simulink model "quad_ndi_test"  (R2017b)
settings: Solver=FixedStepDiscrete  StartTime=0.0  StopTime=10  FixedStep=0.004  RelTol=1e-3
undefined symbols (not defined in the file or in its folder): DiscIntNeverNeededParam
libraries: simulink x3
settings Model: Creator=marcell  LastModifiedBy=max
settings DataIOCC: LimitDataPoints=on
settings OptimizationCC: DefaultParameterBehavior=Inlined  UseFloatMulNetSlope=on  DefaultUnderspecifiedDataType=single  InlineInvariantSignals=on  PassReuseOutputArgsAs=Individual arguments  ZeroExternalMemoryAtStartup=off  ZeroInternalMemoryAtStartup=off  NoFixptDivByZeroProtection=on  EfficientFloat2IntCast=on  LifeSpan=1
settings DebuggingCC: AllowSymbolicDim=off  SFUnexpectedBacktrackingDiag=warning  SFNoUnconditionalDefaultTransitionDiag=warning  SFExecutionAtInitializationDiag=none
settings HardwareCC: ProdBitPerPointer=32  ProdBitPerSizeT=32  ProdBitPerPtrDiffT=32  ProdLargestAtomicInteger=Long  ProdLargestAtomicFloat=Double  ProdWordSize=32  ProdHWDeviceType=ARM Compatible->ARM Cortex
settings ModelReferenceCC: PropagateSignalLabelsOutOfModel=off
settings SFSimCC: MATLABDynamicMemAlloc=off
settings RTWCC: SystemTargetFile=ert.tlc  GenCodeOnly=on  TemplateMakefile=ert_default_tmf  GenerateReport=on  IncludeHyperlinkInReport=on  LaunchReport=on  TargetLang=C++  GenerateTraceInfo=on  GenerateTraceReport=on  GenerateTraceReportSl=on  GenerateTraceReportSf=on  GenerateTraceReportEml=on
settings CodeAppCC: ForceParamTrailComments=on  IgnoreCustomStorageClasses=off  SimulinkDataObjDesc=on  CustomSymbolStrGlobalVar=rt$N$M  CustomSymbolStrType=$N$M  CustomSymbolStrFcn=$N$M$F  CustomSymbolStrMacro=$N$M  InsertBlockDesc=on  StateflowObjectComments=on
settings ERTTargetCC: MultiwordLength=2048  GenerateSampleERTMain=on  IncludeMdlTerminateFcn=off  CombineSignalStateStructs=on  SupportAbsoluteTime=off  MultiInstanceERTCode=on  CodeInterfacePackaging=C++ class  SupportNonFinite=off  SupportComplex=off  SupportNonInlinedSFcns=on  InlinedParameterPlacement=NonHierarchical  RootIOFormat=Structure reference  ERTCustomFileTemplate=example_file_process.tlc  ERTFilePackagingFormat=CompactWithDataFile  ConvertIfToSwitch=off  SuppressUnreachableDefaultCases=off
settings ConfigComp: CovMetricSettings=dw  CovHtmlReporting=on  CovSaveCumulativeToWorkspaceVar=on  CovSaveSingleToWorkspaceVar=on  CovExternalEMLEnable=off

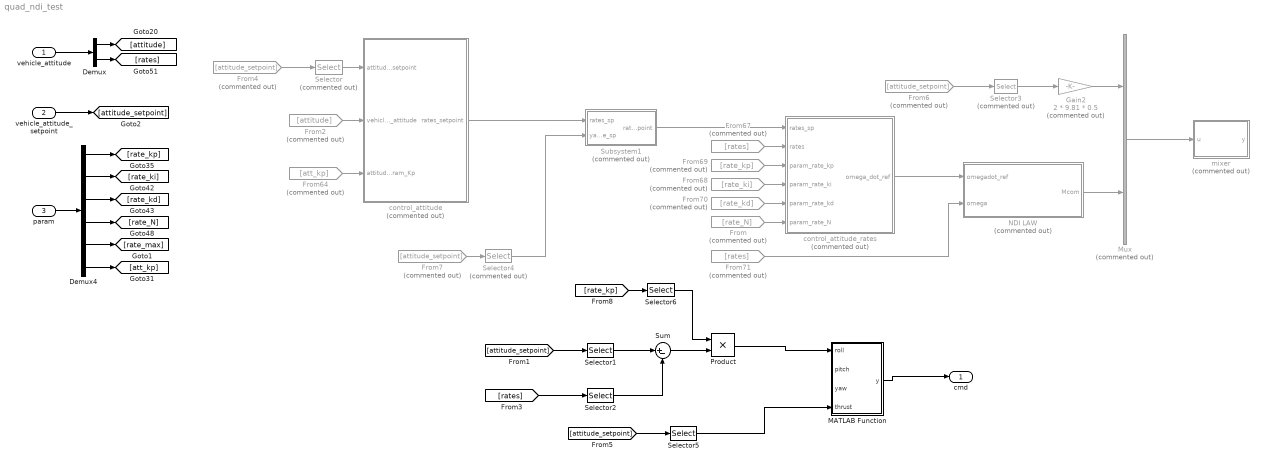
== system quad_ndi_test ==
  vehicle_attitude : Inport  OutDataTypeStr=single  PortDimensions=6
  vehicle_attitude_setpoint : Inport  Port=2  OutDataTypeStr=single  PortDimensions=4
  param : Inport  Port=3  OutDataTypeStr=single  PortDimensions=18
  Demux : Demux  Outputs=[3 3]
  Demux4 : Demux  Outputs=[3 3 3 3 3 3]
  From : From  Commented=on  GotoTag=rate_N
  From2 : From  Commented=on  GotoTag=attitude
  From4 : From  Commented=on  GotoTag=attitude_setpoint
  From6 : From  Commented=on  GotoTag=attitude_setpoint
  From64 : From  Commented=on  GotoTag=att_kp
  From67 : From  Commented=on  GotoTag=rates
  From68 : From  Commented=on  GotoTag=rate_ki
  From69 : From  Commented=on  GotoTag=rate_kp
  From7 : From  Commented=on  GotoTag=attitude_setpoint
  From70 : From  Commented=on  GotoTag=rate_kd
  From71 : From  Commented=on  GotoTag=rates
  Gain2 : Gain  Commented=on  Gain=2 * 9.81 * 0.5
  MATLAB Function : MATLAB Function  TreatAsAtomicUnit=on
  Mux : Mux  Commented=on  Inputs=[1 3]
  NDI LAW : MATLAB Function  Commented=on  TreatAsAtomicUnit=on
  Product : Product
  Selector : Selector  Commented=on  InputPortWidth=4  IndexOptions=Index vector (dialog)  Indices=1:3  OutputSizes=1
  Selector1 : Selector  InputPortWidth=4  IndexOptions=Index vector (dialog)  Indices=1  OutputSizes=1
  Selector2 : Selector  InputPortWidth=3  IndexOptions=Index vector (dialog)  Indices=1  OutputSizes=1
  Selector3 : Selector  Commented=on  InputPortWidth=4  IndexOptions=Index vector (dialog)  Indices=4  OutputSizes=1
  Selector4 : Selector  Commented=on  InputPortWidth=4  IndexOptions=Index vector (dialog)  Indices=3  OutputSizes=1
  Selector5 : Selector  InputPortWidth=4  IndexOptions=Index vector (dialog)  Indices=4  OutputSizes=1
  Selector6 : Selector  InputPortWidth=3  IndexOptions=Index vector (dialog)  Indices=1  OutputSizes=1
  Subsystem1 : Subsystem  Commented=on
  Sum : Sum  Inputs=|+-
  control_attitude : Subsystem  Commented=on  TreatAsAtomicUnit=on
  control_attitude_rates : Subsystem  Commented=on  TreatAsAtomicUnit=on
  mixer : MATLAB Function  Commented=on  TreatAsAtomicUnit=on
  cmd : Outport
  wires:
  vehicle_attitude/1 -> Demux/1
  Demux/1 -> [attitude]
  Demux4/1 -> [rate_kp]
  Demux4/2 -> [rate_ki]
  Demux4/3 -> [rate_kd]
  Demux4/4 -> [rate_N]
  From6/1 -> Selector3/1
  NDI LAW/1(Mcom) -> Mux/2
  control_attitude_rates/1(omega_dot_ref) -> NDI LAW/1(omegadot_ref)
  From2/1 -> control_attitude/2(vehicle_attitude)
  From64/1 -> control_attitude/3(attitude_param_Kp)
  From70/1 -> control_attitude_rates/5(param_rate_kd)
  control_attitude/1(rates_setpoint) -> Subsystem1/1(rates_sp)
  Subsystem1/1(rates_setpoint) -> control_attitude_rates/1(rates_sp)
  From67/1 -> control_attitude_rates/2(rates)
  From68/1 -> control_attitude_rates/4(param_rate_ki)
  From69/1 -> control_attitude_rates/3(param_rate_kp)
  From71/1 -> NDI LAW/2(omega)
  From/1 -> control_attitude_rates/6(param_rate_N)
  Selector3/1 -> Gain2/1
  Mux/1 -> mixer/1(u)
  param/1 -> Demux4/1
  Demux4/5 -> [rate_max]
  Demux4/6 -> [att_kp]
  Demux/2 -> [rates]
  vehicle_attitude_setpoint/1 -> [attitude_setpoint]
  From4/1 -> Selector/1
  Selector/1 -> control_attitude/1(attitude_setpoint)
  From7/1 -> Selector4/1
  Selector4/1 -> Subsystem1/2(yawrate_sp)
  Gain2/1 -> Mux/1
  [attitude_setpoint] -> Selector1/1
  [rates] -> Selector2/1
  Selector1/1 -> Sum/1
  Selector2/1 -> Sum/2
  Sum/1 -> Product/2
  Product/1 -> MATLAB Function/1(roll)
  MATLAB Function/1(y) -> cmd/1
  [attitude_setpoint] -> Selector5/1
  Selector5/1 -> MATLAB Function/4(thrust)
  [rate_kp] -> Selector6/1
  Selector6/1 -> Product/1

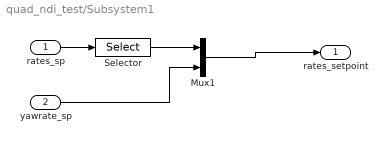
== system quad_ndi_test/Subsystem1 ==
  rates_sp : Inport
  yawrate_sp : Inport  Port=2
  Mux1 : Mux  Inputs=[2 1]
  Selector : Selector  InputPortWidth=3  IndexOptions=Index vector (dialog)  Indices=1:2  OutputSizes=1
  rates_setpoint : Outport
  wires:
  Mux1/1 -> rates_setpoint/1
  rates_sp/1 -> Selector/1
  Selector/1 -> Mux1/1
  yawrate_sp/1 -> Mux1/2

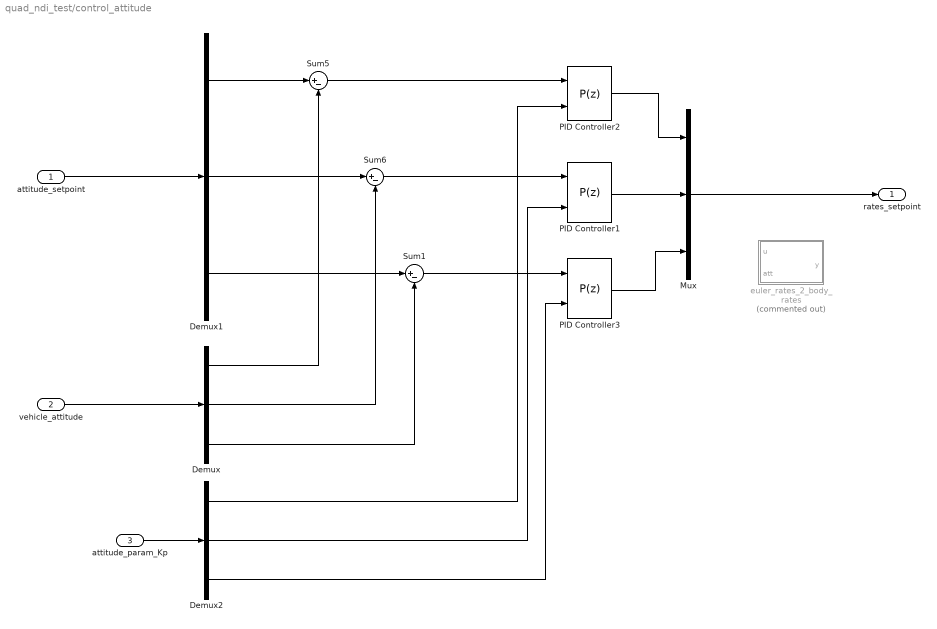
== system quad_ndi_test/control_attitude ==
  attitude_setpoint : Inport
  vehicle_attitude : Inport  Port=2
  attitude_param_Kp : Inport  Port=3
  Demux : Demux  Outputs=3
  Demux1 : Demux  Outputs=3
  Demux2 : Demux  Outputs=3
  Mux : Mux  Inputs=3
  PID Controller1 : simulink/Continuous/PID Controller  Controller=P  TimeDomain=Discrete-time  SampleTime=-1  IntegratorMethod=Forward Euler  FilterMethod=Forward Euler  Form=Parallel  UseFilter=on  ControllerParametersSource=external  P=1/0.3  I=0  D=0  N=100  InitialConditionSource=internal  InitialConditionForIntegrator=0  InitialConditionForFilter=0  ExternalReset=none  LimitOutput=off  UpperSaturationLimit=inf  LowerSaturationLimit=-inf  LinearizeAsGain=on  AntiWindupMode=none  Kb=1  TrackingMode=off  Kt=1  PParamMin=[]  PParamMax=[]  PParamDataTypeStr=single  IParamMin=[]  IParamMax=[]  IParamDataTypeStr=single  DParamMin=[]  DParamMax=[]  NParamMin=[]  NParamMax=[]  KbParamMin=[]  KbParamMax=[]  KtParamMin=[]  KtParamMax=[]  POutMin=[]  POutMax=[]  POutDataTypeStr=single  PGainOutDataTypeStr=single  PProdOutDataTypeStr=single  IOutMin=[]  IOutMax=[]  IOutDataTypeStr=single  IGainOutDataTypeStr=single  IProdOutDataTypeStr=single  DOutMin=[]  DOutMax=[]  NOutMin=[]  NOutMax=[]  KbOutMin=[]  KbOutMax=[]  KtOutMin=[]  KtOutMax=[]  IntegratorOutMin=[]  IntegratorOutMax=[]  FilterOutMin=[]  FilterOutMax=[]  SumOutMin=[]  SumOutMax=[]  SumOutDataTypeStr=single  SumI1OutMin=[]  SumI1OutMax=[]  SumI2OutMin=[]  SumI2OutMax=[]  SumI3OutMin=[]  SumI3OutMax=[]  SumDOutMin=[]  SumDOutMax=[]  SumAccumDataTypeStr=single  SaturationOutMin=[]  SaturationOutMax=[]  IntegratorContinuousStateAttributes=''  IntegratorStateMustResolveToSignalObject=off  IntegratorRTWStateStorageClass=Auto  FilterContinuousStateAttributes=''  FilterStateMustResolveToSignalObject=off  FilterRTWStateStorageClass=Auto  DifferentiatorICPrevScaledInput=0  DifferentiatorOutMin=[]  DifferentiatorOutMax=[]  InitialConditionSetting=State (most efficient)  FilterDiffOutCoefMin=[]  FilterDiffOutCoefMax=[]  SumDenOutMin=[]  SumDenOutMax=[]  SumNumOutMin=[]  SumNumOutMax=[]  ReciprocalOutMin=[]  ReciprocalOutMax=[]  DivideOutMin=[]  DivideOutMax=[]  TunerSelectOption=Transfer Function Based (PID Tuner App)
  PID Controller2 : simulink/Continuous/PID Controller  Controller=P  TimeDomain=Discrete-time  SampleTime=-1  IntegratorMethod=Forward Euler  FilterMethod=Forward Euler  Form=Parallel  UseFilter=on  ControllerParametersSource=external  P=1/0.3  I=0  D=0  N=100  InitialConditionSource=internal  InitialConditionForIntegrator=0  InitialConditionForFilter=0  ExternalReset=none  LimitOutput=off  UpperSaturationLimit=inf  LowerSaturationLimit=-inf  LinearizeAsGain=on  AntiWindupMode=none  Kb=1  TrackingMode=off  Kt=1  PParamMin=[]  PParamMax=[]  PParamDataTypeStr=single  IParamMin=[]  IParamMax=[]  IParamDataTypeStr=single  DParamMin=[]  DParamMax=[]  NParamMin=[]  NParamMax=[]  KbParamMin=[]  KbParamMax=[]  KtParamMin=[]  KtParamMax=[]  POutMin=[]  POutMax=[]  POutDataTypeStr=single  PGainOutDataTypeStr=single  PProdOutDataTypeStr=single  IOutMin=[]  IOutMax=[]  IOutDataTypeStr=single  IGainOutDataTypeStr=single  IProdOutDataTypeStr=single  DOutMin=[]  DOutMax=[]  NOutMin=[]  NOutMax=[]  KbOutMin=[]  KbOutMax=[]  KtOutMin=[]  KtOutMax=[]  IntegratorOutMin=[]  IntegratorOutMax=[]  FilterOutMin=[]  FilterOutMax=[]  SumOutMin=[]  SumOutMax=[]  SumOutDataTypeStr=single  SumI1OutMin=[]  SumI1OutMax=[]  SumI2OutMin=[]  SumI2OutMax=[]  SumI3OutMin=[]  SumI3OutMax=[]  SumDOutMin=[]  SumDOutMax=[]  SumAccumDataTypeStr=single  SaturationOutMin=[]  SaturationOutMax=[]  IntegratorContinuousStateAttributes=''  IntegratorStateMustResolveToSignalObject=off  IntegratorRTWStateStorageClass=Auto  FilterContinuousStateAttributes=''  FilterStateMustResolveToSignalObject=off  FilterRTWStateStorageClass=Auto  DifferentiatorICPrevScaledInput=0  DifferentiatorOutMin=[]  DifferentiatorOutMax=[]  InitialConditionSetting=State (most efficient)  FilterDiffOutCoefMin=[]  FilterDiffOutCoefMax=[]  SumDenOutMin=[]  SumDenOutMax=[]  SumNumOutMin=[]  SumNumOutMax=[]  ReciprocalOutMin=[]  ReciprocalOutMax=[]  DivideOutMin=[]  DivideOutMax=[]  TunerSelectOption=Transfer Function Based (PID Tuner App)
  PID Controller3 : simulink/Continuous/PID Controller  Controller=P  TimeDomain=Discrete-time  SampleTime=-1  IntegratorMethod=Forward Euler  FilterMethod=Forward Euler  Form=Parallel  UseFilter=on  ControllerParametersSource=external  P=1/0.3  I=0  D=0  N=100  InitialConditionSource=internal  InitialConditionForIntegrator=0  InitialConditionForFilter=0  ExternalReset=none  LimitOutput=off  UpperSaturationLimit=inf  LowerSaturationLimit=-inf  LinearizeAsGain=on  AntiWindupMode=none  Kb=1  TrackingMode=off  Kt=1  PParamMin=[]  PParamMax=[]  PParamDataTypeStr=single  IParamMin=[]  IParamMax=[]  IParamDataTypeStr=single  DParamMin=[]  DParamMax=[]  NParamMin=[]  NParamMax=[]  KbParamMin=[]  KbParamMax=[]  KtParamMin=[]  KtParamMax=[]  POutMin=[]  POutMax=[]  POutDataTypeStr=single  PGainOutDataTypeStr=single  PProdOutDataTypeStr=single  IOutMin=[]  IOutMax=[]  IOutDataTypeStr=single  IGainOutDataTypeStr=single  IProdOutDataTypeStr=single  DOutMin=[]  DOutMax=[]  NOutMin=[]  NOutMax=[]  KbOutMin=[]  KbOutMax=[]  KtOutMin=[]  KtOutMax=[]  IntegratorOutMin=[]  IntegratorOutMax=[]  FilterOutMin=[]  FilterOutMax=[]  SumOutMin=[]  SumOutMax=[]  SumOutDataTypeStr=single  SumI1OutMin=[]  SumI1OutMax=[]  SumI2OutMin=[]  SumI2OutMax=[]  SumI3OutMin=[]  SumI3OutMax=[]  SumDOutMin=[]  SumDOutMax=[]  SumAccumDataTypeStr=single  SaturationOutMin=[]  SaturationOutMax=[]  IntegratorContinuousStateAttributes=''  IntegratorStateMustResolveToSignalObject=off  IntegratorRTWStateStorageClass=Auto  FilterContinuousStateAttributes=''  FilterStateMustResolveToSignalObject=off  FilterRTWStateStorageClass=Auto  DifferentiatorICPrevScaledInput=0  DifferentiatorOutMin=[]  DifferentiatorOutMax=[]  InitialConditionSetting=State (most efficient)  FilterDiffOutCoefMin=[]  FilterDiffOutCoefMax=[]  SumDenOutMin=[]  SumDenOutMax=[]  SumNumOutMin=[]  SumNumOutMax=[]  ReciprocalOutMin=[]  ReciprocalOutMax=[]  DivideOutMin=[]  DivideOutMax=[]  TunerSelectOption=Transfer Function Based (PID Tuner App)
  Sum1 : Sum  Inputs=|+-
  Sum5 : Sum  Inputs=|+-
  Sum6 : Sum  Inputs=|+-
  euler_rates_2_body_rates : MATLAB Function  Commented=on  TreatAsAtomicUnit=on
  rates_setpoint : Outport
  wires:
  Sum5/1 -> PID Controller2/1
  Sum6/1 -> PID Controller1/1
  Sum1/1 -> PID Controller3/1
  Demux/1 -> Sum5/2
  Demux/2 -> Sum6/2
  Demux/3 -> Sum1/2
  vehicle_attitude/1 -> Demux/1
  attitude_setpoint/1 -> Demux1/1
  Demux1/1 -> Sum5/1
  Demux1/2 -> Sum6/1
  Demux1/3 -> Sum1/1
  attitude_param_Kp/1 -> Demux2/1
  Demux2/1 -> PID Controller2/2
  Demux2/2 -> PID Controller1/2
  Demux2/3 -> PID Controller3/2
  PID Controller2/1 -> Mux/1
  PID Controller1/1 -> Mux/2
  PID Controller3/1 -> Mux/3
  Mux/1 -> rates_setpoint/1

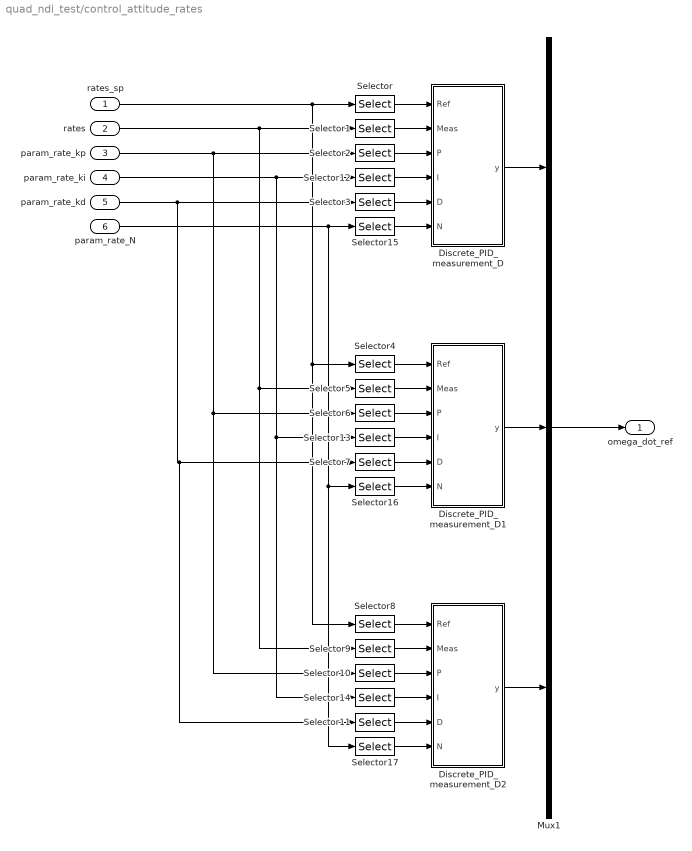
== system quad_ndi_test/control_attitude_rates ==
  rates_sp : Inport
  rates : Inport  Port=2
  param_rate_kp : Inport  Port=3
  param_rate_ki : Inport  Port=4
  param_rate_kd : Inport  Port=5
  param_rate_N : Inport  Port=6
  Discrete_PID_measurement_D : Subsystem
  Discrete_PID_measurement_D1 : Subsystem
  Discrete_PID_measurement_D2 : Subsystem
  Mux1 : Mux  Inputs=3
  Selector{,1..3,12,15} (6 alike) : Selector  InputPortWidth=3  IndexOptions=Index vector (dialog)  Indices=1  OutputSizes=1
  Selector{8..11,14} (5 alike) : Selector  InputPortWidth=3  IndexOptions=Index vector (dialog)  Indices=3  OutputSizes=1
  Selector{4..7,13,16..17} (7 alike) : Selector  InputPortWidth=3  IndexOptions=Index vector (dialog)  Indices=2  OutputSizes=1
  omega_dot_ref : Outport
  wires:
  Mux1/1 -> omega_dot_ref/1
  Discrete_PID_measurement_D/1(y) -> Mux1/1
  Discrete_PID_measurement_D1/1(y) -> Mux1/2
  Discrete_PID_measurement_D2/1(y) -> Mux1/3
  Selector17/1 -> Discrete_PID_measurement_D2/6(N)
  Selector16/1 -> Discrete_PID_measurement_D1/6(N)
  Selector15/1 -> Discrete_PID_measurement_D/6(N)
  Selector3/1 -> Discrete_PID_measurement_D/5(D)
  Selector2/1 -> Discrete_PID_measurement_D/3(P)
  Selector1/1 -> Discrete_PID_measurement_D/2(Meas)
  Selector/1 -> Discrete_PID_measurement_D/1(Ref)
  Selector4/1 -> Discrete_PID_measurement_D1/1(Ref)
  Selector5/1 -> Discrete_PID_measurement_D1/2(Meas)
  Selector6/1 -> Discrete_PID_measurement_D1/3(P)
  Selector7/1 -> Discrete_PID_measurement_D1/5(D)
  rates_sp/1 -> Selector8/1, Selector4/1, Selector/1
  Selector10/1 -> Discrete_PID_measurement_D2/3(P)
  Selector9/1 -> Discrete_PID_measurement_D2/2(Meas)
  Selector8/1 -> Discrete_PID_measurement_D2/1(Ref)
  Selector11/1 -> Discrete_PID_measurement_D2/5(D)
  rates/1 -> Selector9/1, Selector5/1, Selector1/1
  param_rate_kp/1 -> Selector6/1, Selector10/1, Selector2/1
  param_rate_kd/1 -> Selector11/1, Selector7/1, Selector3/1
  Selector12/1 -> Discrete_PID_measurement_D/4(I)
  Selector13/1 -> Discrete_PID_measurement_D1/4(I)
  Selector14/1 -> Discrete_PID_measurement_D2/4(I)
  param_rate_ki/1 -> Selector13/1, Selector14/1, Selector12/1
  param_rate_N/1 -> Selector17/1, Selector16/1, Selector15/1

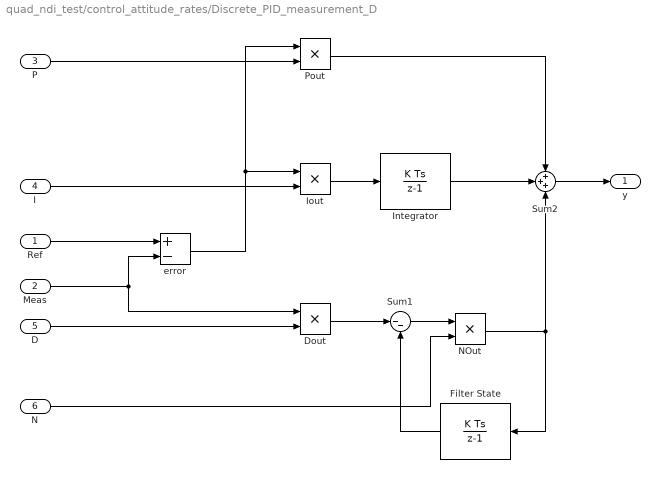
== system quad_ndi_test/control_attitude_rates/Discrete_PID_measurement_D ==
  Ref : Inport
  Meas : Inport  Port=2
  P : Inport  Port=3
  I : Inport  Port=4
  D : Inport  Port=5
  N : Inport  Port=6
  Dout : Product  OutDataTypeStr=single
  Filter State : DiscreteIntegrator  InitialConditionSetting=State (most efficient)  SampleTime=-1  OutDataTypeStr=single  ICPrevOutput=DiscIntNeverNeededParam  ICPrevScaledInput=DiscIntNeverNeededParam
  Integrator : DiscreteIntegrator  InitialConditionSetting=State (most efficient)  SampleTime=-1  OutDataTypeStr=single  ICPrevOutput=DiscIntNeverNeededParam  ICPrevScaledInput=DiscIntNeverNeededParam
  Iout : Product  OutDataTypeStr=single
  NOut : Product  OutDataTypeStr=single
  Pout : Product  OutDataTypeStr=single
  Sum1 : Sum  Inputs=|--
  Sum2 : Sum  Inputs=+++
  error : Sum  Inputs=+-
  y : Outport  InitialOutput=0
  wires:
  Iout/1 -> Integrator/1
  Integrator/1 -> Sum2/2
  Dout/1 -> Sum1/1
  Sum1/1 -> NOut/1
  NOut/1 -> Filter State/1, Sum2/3
  Filter State/1 -> Sum1/2
  Pout/1 -> Sum2/1
  Sum2/1 -> y/1
  P/1 -> Pout/2
  I/1 -> Iout/2
  D/1 -> Dout/2
  N/1 -> NOut/2
  Ref/1 -> error/1
  error/1 -> Pout/1, Iout/1
  Meas/1 -> error/2, Dout/1

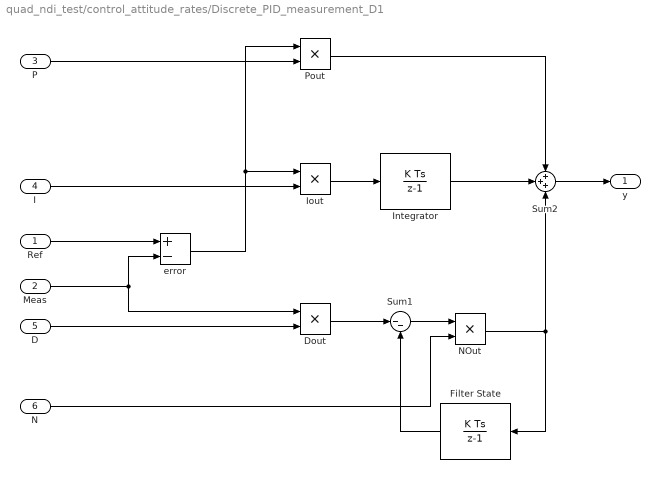
== system quad_ndi_test/control_attitude_rates/Discrete_PID_measurement_D1 ==
  Ref : Inport
  Meas : Inport  Port=2
  P : Inport  Port=3
  I : Inport  Port=4
  D : Inport  Port=5
  N : Inport  Port=6
  Dout : Product  OutDataTypeStr=single
  Filter State : DiscreteIntegrator  InitialConditionSetting=State (most efficient)  SampleTime=-1  OutDataTypeStr=single  ICPrevOutput=DiscIntNeverNeededParam  ICPrevScaledInput=DiscIntNeverNeededParam
  Integrator : DiscreteIntegrator  InitialConditionSetting=State (most efficient)  SampleTime=-1  OutDataTypeStr=single  ICPrevOutput=DiscIntNeverNeededParam  ICPrevScaledInput=DiscIntNeverNeededParam
  Iout : Product  OutDataTypeStr=single
  NOut : Product  OutDataTypeStr=single
  Pout : Product  OutDataTypeStr=single
  Sum1 : Sum  Inputs=|--
  Sum2 : Sum  Inputs=+++
  error : Sum  Inputs=+-
  y : Outport  InitialOutput=0
  wires:
  Meas/1 -> Dout/1, error/2
  error/1 -> Iout/1, Pout/1
  Ref/1 -> error/1
  N/1 -> NOut/2
  D/1 -> Dout/2
  I/1 -> Iout/2
  P/1 -> Pout/2
  Sum2/1 -> y/1
  Pout/1 -> Sum2/1
  Filter State/1 -> Sum1/2
  NOut/1 -> Sum2/3, Filter State/1
  Sum1/1 -> NOut/1
  Dout/1 -> Sum1/1
  Integrator/1 -> Sum2/2
  Iout/1 -> Integrator/1

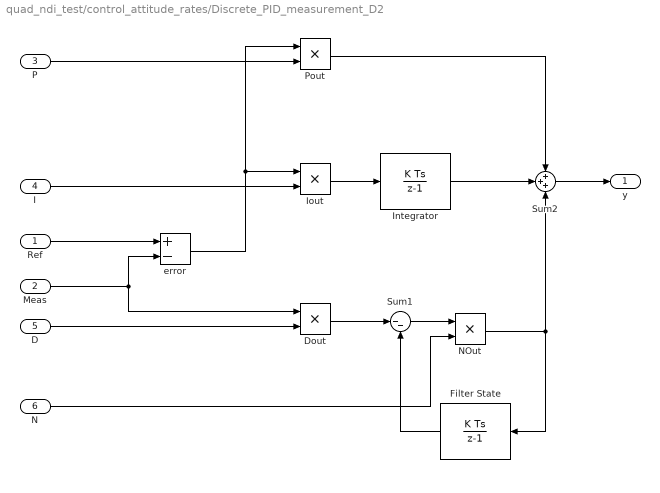
== system quad_ndi_test/control_attitude_rates/Discrete_PID_measurement_D2 ==
  Ref : Inport
  Meas : Inport  Port=2
  P : Inport  Port=3
  I : Inport  Port=4
  D : Inport  Port=5
  N : Inport  Port=6
  Dout : Product  OutDataTypeStr=single
  Filter State : DiscreteIntegrator  InitialConditionSetting=State (most efficient)  SampleTime=-1  OutDataTypeStr=single  ICPrevOutput=DiscIntNeverNeededParam  ICPrevScaledInput=DiscIntNeverNeededParam
  Integrator : DiscreteIntegrator  InitialConditionSetting=State (most efficient)  SampleTime=-1  OutDataTypeStr=single  ICPrevOutput=DiscIntNeverNeededParam  ICPrevScaledInput=DiscIntNeverNeededParam
  Iout : Product  OutDataTypeStr=single
  NOut : Product  OutDataTypeStr=single
  Pout : Product  OutDataTypeStr=single
  Sum1 : Sum  Inputs=|--
  Sum2 : Sum  Inputs=+++
  error : Sum  Inputs=+-
  y : Outport  InitialOutput=0
  wires:
  Iout/1 -> Integrator/1
  Integrator/1 -> Sum2/2
  Dout/1 -> Sum1/1
  Sum1/1 -> NOut/1
  NOut/1 -> Filter State/1, Sum2/3
  Filter State/1 -> Sum1/2
  Pout/1 -> Sum2/1
  Sum2/1 -> y/1
  P/1 -> Pout/2
  I/1 -> Iout/2
  D/1 -> Dout/2
  N/1 -> NOut/2
  Ref/1 -> error/1
  error/1 -> Pout/1, Iout/1
  Meas/1 -> error/2, Dout/1

== matlab function quad_ndi_test/MATLAB Function ==
  data: roll input; y output; pitch input; yaw input; thrust input
function y = fcn(roll,pitch,yaw,thrust)


mot1 = ((-roll+pitch)/2 -yaw/4) * thust;


y = u;

== matlab function quad_ndi_test/mixer ==
  data: u input; y output
function y = fcn(u)
%#codegen
k = 4.5; % max motor thrust
L  = 0.0707; % arm length
kMT = 0.01; % max motor moment
Fmat = [k  k   k   k];    % Fzb
Mmat = [ -L*k    L*k  L*k    -L*k;          % roll moment
         L*k    -L*k  +L*k    -L*k;          % pitch moment
         kMT*k   kMT*k -kMT*k  -kMT*k];       % yaw momentMmat = [ -L*k(1)    L*k(2)  L*k(3)    -L*k(4);          % roll moment
Tmn2 = [Fmat;Mmat];
Tnm2 = pinv(Tmn2);
y = Tnm2 * u;

== matlab function quad_ndi_test/control_attitude/euler_rates_2_body_rates ==
  data: u input; y output; att input
function y = fcn(u,att)
%#codegen
phi   =	att(1); 
theta =	att(2);
% Frequently used functions
sphi = sin(phi);   cphi = cos(phi);
sthe = sin(theta); cthe = cos(theta);
if abs(cthe)<=single(0.00001)  % Hack to avoid singulariy at +/- pi/2
  cthe = single(0.00001) * sign(cthe);
end
% Euler Rates to Body Rates:    
Hbe  = [1,  0,    -sthe;
        0,  cphi,  sphi*cthe;
        0  -sphi,  cphi*cthe];
y = Hbe * u;

== matlab function quad_ndi_test/NDI LAW ==
  data: omegadot_ref input; Mcom output; omega input
function Mcom = fcn(omegadot_ref,omega)
% NDI control Law
Ib = single(diag([0.002,0.002,0.003]));
Mcom = Ib * omegadot_ref + cross(omega, Ib * omega);
